simulink model "PV1"  (R2024b)
settings: Solver=ode4  StartTime=0.0  StopTime=100  FixedStep=0.00002  RelTol=1e-3
undefined symbols (not defined in the file): Ion, Lithium
libraries: spsSeriesRLCBranchLib x10, spsDiodeLib x3, spsMosfetLib x3, simulink x3, spsVoltageMeasurementLib x3, spsPVArrayLib x3, spsBatteryLib x1, spspowerguiLib x1
settings Model: Creator=Admin  LastModifiedBy=govin
settings RTWCC: GPUComputeCapability=3.5

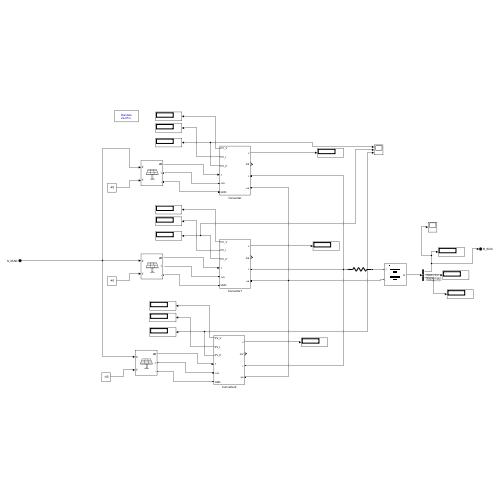
[thumbnail: Simulink's stored preview of the top-level diagram]
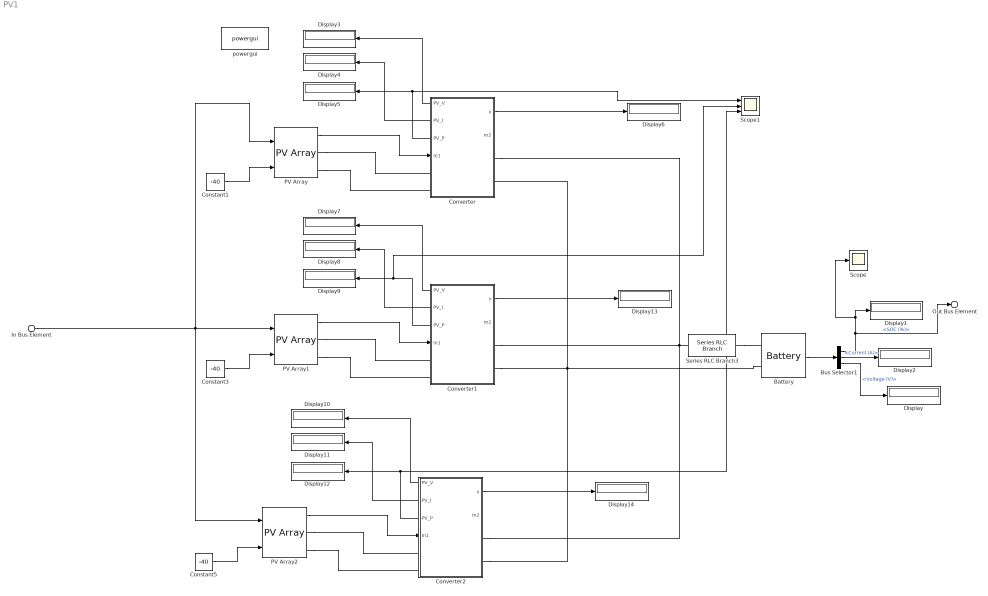
== system PV1 ==
  In Bus Element : Inport  PortName=S_IRAD
  Battery : spsBatteryLib/Battery  BatType=Lithium-Ion  NomV=8.4  NomQ=8  SOC=30  Batt_Tr=1  PresetModel=on  MaxQ=8  MinV=6.3  FullV=9.7775  Dis_rate=3.4783  R=0.0105  Normal_OP=7.2348  expZone="[9.0752     0.39304]"
  Bus Selector1 : BusSelector  OutputSignals=SOC (%),Current (A),Voltage (V)
  Constant1 : Constant  Value=-40
  Constant3 : Constant  Value=-40
  Constant5 : Constant  Value=-40
  Converter : Subsystem
      settings: PortSchema="{\"entries\":[{\"content\":{\"sides\":[{\"content\":{\"connectorIds\":[\"Out3\",\"Out4\",\"Out5\",\"In1\",\"LConn1\",\"LConn2\"]},\"type\":\"ConnectorPlacement.EquallySpacedRectSide\",\"uuid\":\"a132338a-6d9d-431e-bfe8-8757d124dffa\"},{\"content\":{\"connectorIds\":[\"Out1\",\"Out2\",\"RConn1\",\"RConn2\"],\"side\":\"RIGHT\"},\"type\":\"ConnectorPlacement.EquallySpacedRectSide\",\"uuid\":\"d50e3670-6251-4d2a-bf58-0033f338dba0\"},{\"content\":{\"side\":\"TOP\"},\"type\":\"ConnectorPlacement.EquallySpacedRectSide\",\"uuid\":\"35bc6587-48f1-421a-8d61-ff55cf247e3f\"}]},\"type\":\"ConnectorPlacement.EquallySpacedConnector\",\"uuid\":\"b4d66b82-5386-42ac-acc1-5dbc35c09c36\"}],\"packageUris\":[\"http://schema.mathworks.com/mf0/Connector/R2020b\"],\"version\":\"1.0\"}"
  Converter1 : Subsystem
      settings: PortSchema="{\"entries\":[{\"content\":{\"sides\":[{\"content\":{\"connectorIds\":[\"Out3\",\"Out4\",\"Out5\",\"In1\",\"LConn1\",\"LConn2\"]},\"type\":\"ConnectorPlacement.EquallySpacedRectSide\",\"uuid\":\"a132338a-6d9d-431e-bfe8-8757d124dffa\"},{\"content\":{\"connectorIds\":[\"Out1\",\"Out2\",\"RConn1\",\"RConn2\"],\"side\":\"RIGHT\"},\"type\":\"ConnectorPlacement.EquallySpacedRectSide\",\"uuid\":\"d50e3670-6251-4d2a-bf58-0033f338dba0\"},{\"content\":{\"side\":\"TOP\"},\"type\":\"ConnectorPlacement.EquallySpacedRectSide\",\"uuid\":\"35bc6587-48f1-421a-8d61-ff55cf247e3f\"}]},\"type\":\"ConnectorPlacement.EquallySpacedConnector\",\"uuid\":\"b4d66b82-5386-42ac-acc1-5dbc35c09c36\"}],\"packageUris\":[\"http://schema.mathworks.com/mf0/Connector/R2020b\"],\"version\":\"1.0\"}"
  Converter2 : Subsystem
      settings: PortSchema="{\"entries\":[{\"content\":{\"sides\":[{\"content\":{\"connectorIds\":[\"Out3\",\"Out4\",\"Out5\",\"In1\",\"LConn1\",\"LConn2\"]},\"type\":\"ConnectorPlacement.EquallySpacedRectSide\",\"uuid\":\"a132338a-6d9d-431e-bfe8-8757d124dffa\"},{\"content\":{\"connectorIds\":[\"Out1\",\"Out2\",\"RConn1\",\"RConn2\"],\"side\":\"RIGHT\"},\"type\":\"ConnectorPlacement.EquallySpacedRectSide\",\"uuid\":\"d50e3670-6251-4d2a-bf58-0033f338dba0\"},{\"content\":{\"side\":\"TOP\"},\"type\":\"ConnectorPlacement.EquallySpacedRectSide\",\"uuid\":\"35bc6587-48f1-421a-8d61-ff55cf247e3f\"}]},\"type\":\"ConnectorPlacement.EquallySpacedConnector\",\"uuid\":\"b4d66b82-5386-42ac-acc1-5dbc35c09c36\"}],\"packageUris\":[\"http://schema.mathworks.com/mf0/Connector/R2020b\"],\"version\":\"1.0\"}"
  Display{,1..14} (15 alike) : Display
  PV Array : spsPVArrayLib/PV Array  Npar=1  Nser=1  PlotType=array @ 25 deg.C & specified irradiances  S_vec="[ 1000  500  100 ]"  Temp_C_vec="[ 45 25  ]"  ModuleName=User-defined  PlotWhenSelected=off  Pm=8.6265  Ncell=7  Voc=19.25  Isc=0.521  Vm=17.15  Im=0.503  beta_Voc_pc=-0.59  alpha_Isc_pc=0.44  beta_Voc=-0.11357  alpha_Isc=0.0022924  IL=0.52617  I0=1.5749e-15  nI=3  Rsh=1905.5562  Rs=0.00066309  RobustModel=off  RobustCellTemperature=313.3991  BAL=on  Tc=1e-6  Tfilter=5e-5
  PV Array1 : spsPVArrayLib/PV Array  Npar=1  Nser=1  PlotType=array @ 25 deg.C & specified irradiances  S_vec="[ 1000  500  100 ]"  Temp_C_vec="[ 45 25  ]"  ModuleName=User-defined  PlotWhenSelected=off  Pm=7.3941  Ncell=7  Voc=16.5  Isc=0.521  Vm=14.7  Im=0.503  beta_Voc_pc=-0.59  alpha_Isc_pc=0.44  beta_Voc=-0.09735  alpha_Isc=0.0022924  IL=0.52104  I0=1.6325e-15  nI=2.8682  Rsh=1633.334  Rs=1.5927  RobustModel=off  RobustCellTemperature=313.3991  BAL=on  Tc=1e-6  Tfilter=5e-5
  PV Array2 : spsPVArrayLib/PV Array  Npar=1  Nser=1  PlotType=array @ 25 deg.C & specified irradiances  S_vec="[ 1000  500  100 ]"  Temp_C_vec="[ 45 25  ]"  ModuleName=User-defined  PlotWhenSelected=off  Pm=8.6265  Ncell=7  Voc=19.25  Isc=0.521  Vm=17.15  Im=0.503  beta_Voc_pc=-0.59  alpha_Isc_pc=0.44  beta_Voc=-0.11357  alpha_Isc=0.0022924  IL=0.52617  I0=1.5749e-15  nI=3  Rsh=1905.5562  Rs=0.00066309  RobustModel=off  RobustCellTemperature=313.3991  BAL=on  Tc=1e-6  Tfilter=5e-5
  Scope : Scope
  Scope1 : Scope  NumInputPorts=3
  Series RLC Branch3 : spsSeriesRLCBranchLib/Series RLC Branch  LConnTagsString=__new0  RConnTagsString=__new0  BranchType=R  Resistance=0.0001  Inductance=1e-3  SetiL0=off  InitialCurrent=0  Capacitance=0  Setx0=off  InitialVoltage=0  Measurements=None
  powergui : spspowerguiLib/powergui  Priority=1  SimulationMode=Discrete  SampleTime=0.00002  frequency=60  Iterations=50  frequencyindice=0  Pbase=100e6  ErrMax=1e-4  UnitsV=kV  UnitsW=MW  buscounter=0  FunctionMessages=off  echomessages=off  EnableUseOfTLC=off  CurrentSourceSwitches=off  DisableSnubberDevices=off  DisableRonSwitches=off  DisableVfSwitches=off  DisplayEquations=off  AutomaticDiscreteSolvers=off  SolverType=Tustin/Backward Euler (TBE)  Interpol=off  ExternalGateDelay=off  methode=off  Ts=100  x0status=blocks  SPID=on  SwTol=0  HookPort=off  NonlinearTolerance=1e-4  nMaxIteration=100  ContinueOnMaxIteration=off  RestoreLinks=warning  ResistiveCurrentMeasurement=off  Frange=[0:2:500]  Ylog=off  Xlog=on  ShowGrid=off  save=off  variable=ZData  structure=0  ZoomFFT=off  StartTime=0.0  cycles=1  DisplayStyle=1  fundamental=60  FreqAxis=off  MaxFrequency=1000  frequencyindicesteady=1  RmsSteady=1  display=off
  Out Bus Element : Outport  PortName=B_SOC
  wires:
  Constant1/1 -> PV Array/2
  Battery/1 -> Bus Selector1/1
  Bus Selector1/2 -> Display2/1  "<Current (A)>"
  Bus Selector1/1 -> Out Bus Element/1, Scope/1, Display1/1  "<SOC (%)>"
  Bus Selector1/3 -> Display/1  "<Voltage (V)>"
  Converter/1(v) -> Display6/1
  PV Array/1 -> Converter/1(In1)
  Converter/3(PV_V) -> Display3/1
  Converter/4(PV_I) -> Display4/1
  Converter/5(PV_P) -> Display5/1, Scope1/1
  Constant3/1 -> PV Array1/2
  Converter1/3(PV_V) -> Display7/1
  Converter1/1(v) -> Display13/1
  PV Array1/1 -> Converter1/1(In1)
  Converter1/4(PV_I) -> Display8/1
  Converter1/5(PV_P) -> Scope1/2, Display9/1
  Constant5/1 -> PV Array2/2
  Converter2/3(PV_V) -> Display10/1
  Converter2/1(v) -> Display14/1
  In Bus Element/1 -> PV Array/1, PV Array2/1, PV Array1/1
  PV Array2/1 -> Converter2/1(In1)
  Converter2/4(PV_I) -> Display11/1
  Converter2/5(PV_P) -> Scope1/3, Display12/1
  connections:
  Battery/LConn2 -- Converter/RConn2 -- Converter2/RConn2 -- Converter1/RConn2
  Converter/RConn1 -- Series RLC Branch3/LConn1 -- Converter2/RConn1 -- Converter1/RConn1
  PV Array/RConn1 -- Converter/LConn1
  PV Array/RConn2 -- Converter/LConn2
  PV Array1/RConn2 -- Converter1/LConn2
  PV Array1/RConn1 -- Converter1/LConn1
  PV Array2/RConn2 -- Converter2/LConn2
  PV Array2/RConn1 -- Converter2/LConn1
  Series RLC Branch3/RConn1 -- Battery/LConn1

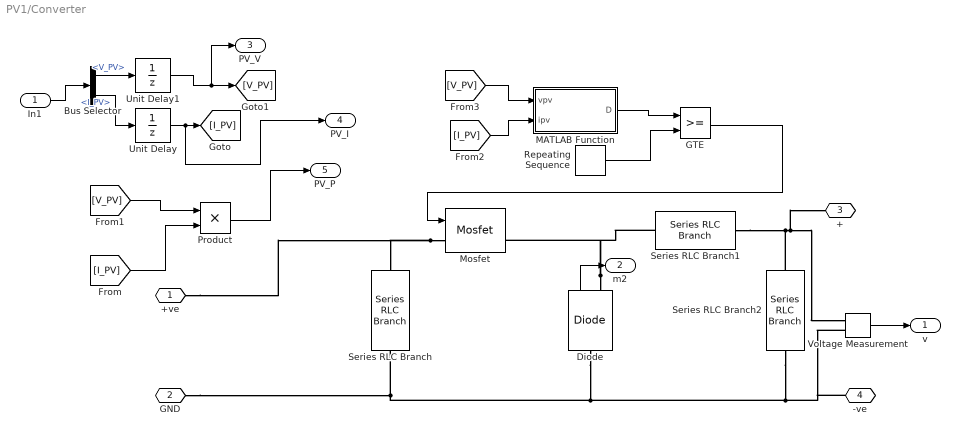
== system PV1/Converter ==
  In1 : Inport
  Bus Selector : BusSelector  OutputSignals=V_PV,I_PV
  Diode : spsDiodeLib/Diode  Ron=0.001  Lon=0  Vf=0.8  IC=0  UseSnubber=0  Rs=500  Cs=250e-9  Measurements=on
  GTE : RelationalOperator  OutDataTypeStr=boolean  RndMeth=Simplest  InputSameDT=off
  MATLAB Function : MATLAB Function  TreatAsAtomicUnit=on
  Mosfet : spsMosfetLib/Mosfet  Ron=0.1  Lon=0  Rd=0.01  Vfd=0  IC=0  Rs=1e5  Cs=inf  Measurements=on
  Product : Product
  Repeating Sequence : simulink/Sources/Repeating Sequence  rep_seq_t=[0 0.0002]  rep_seq_y=[0 1]
  Series RLC Branch : spsSeriesRLCBranchLib/Series RLC Branch  LConnTagsString=__new0  RConnTagsString=__new0  BranchType=RC  Resistance=0.0001  Inductance=1e-3  SetiL0=off  InitialCurrent=0  Capacitance=1000e-6  Setx0=off  InitialVoltage=0  Measurements=None
  Series RLC Branch1 : spsSeriesRLCBranchLib/Series RLC Branch  LConnTagsString=__new0  RConnTagsString=__new0  BranchType=L  Resistance=0.0001  Inductance=8.346e-3  SetiL0=off  InitialCurrent=0  Capacitance=1000e-6  Setx0=off  InitialVoltage=0  Measurements=None
  Series RLC Branch2 : spsSeriesRLCBranchLib/Series RLC Branch  LConnTagsString=__new0  RConnTagsString=__new0  BranchType=C  Resistance=0.0001  Inductance=0.865e-3  SetiL0=off  InitialCurrent=0  Capacitance=30.56e-6  Setx0=off  InitialVoltage=0  Measurements=None
  Unit Delay : UnitDelay  SampleTime=-1  HasFrameUpgradeWarning=on
  Unit Delay1 : UnitDelay  SampleTime=-1  HasFrameUpgradeWarning=on
  Voltage Measurement : spsVoltageMeasurementLib/Voltage Measurement  PhasorSimulation=off  OutputType=Complex  PSBequivalent=0
  +ve : PMIOPort  Side=Left
  GND : PMIOPort  Port=2  Side=Left
  + : PMIOPort  Port=3  Side=Right
  -ve : PMIOPort  Port=4  Side=Right
  v : Outport
  m2 : Outport  Port=2
  PV_V : Outport  Port=3
  PV_I : Outport  Port=4
  PV_P : Outport  Port=5
  wires:
  [V_PV] -> MATLAB Function/1(vpv)
  [I_PV] -> MATLAB Function/2(ipv)
  Repeating Sequence/1 -> GTE/2
  GTE/1 -> Mosfet/1
  MATLAB Function/1(D) -> GTE/1
  Diode/1 -> m2/1
  Voltage Measurement/1 -> v/1
  Bus Selector/2 -> Unit Delay/1  "<I_PV>"
  In1/1 -> Bus Selector/1
  Unit Delay/1 -> PV_I/1, [I_PV]
  Unit Delay1/1 -> PV_V/1, [V_PV]
  Bus Selector/1 -> Unit Delay1/1  "<V_PV>"
  [I_PV] -> Product/2
  [V_PV] -> Product/1
  Product/1 -> PV_P/1
  connections:
  Diode/LConn1 -- Voltage Measurement/LConn2 -- -ve/RConn1 -- Series RLC Branch2/RConn1 -- GND/RConn1 -- Series RLC Branch/RConn1
  Diode/RConn1 -- Series RLC Branch1/LConn1 -- Mosfet/RConn1
  Mosfet/LConn1 -- +ve/RConn1 -- Series RLC Branch/LConn1
  Series RLC Branch1/RConn1 -- Series RLC Branch2/LConn1 -- +/RConn1 -- Voltage Measurement/LConn1

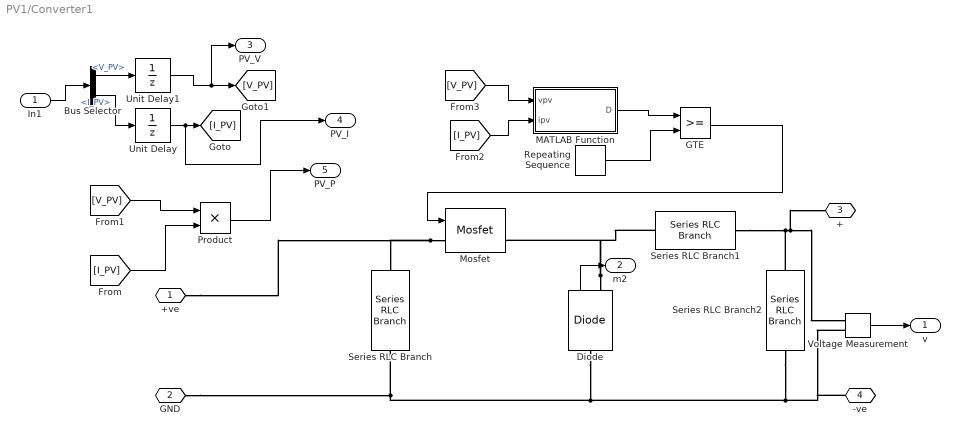
== system PV1/Converter1 ==
  In1 : Inport
  Bus Selector : BusSelector  OutputSignals=V_PV,I_PV
  Diode : spsDiodeLib/Diode  Ron=0.001  Lon=0  Vf=0.8  IC=0  UseSnubber=0  Rs=500  Cs=250e-9  Measurements=on
  GTE : RelationalOperator  OutDataTypeStr=boolean  RndMeth=Simplest  InputSameDT=off
  MATLAB Function : MATLAB Function  TreatAsAtomicUnit=on
  Mosfet : spsMosfetLib/Mosfet  Ron=0.1  Lon=0  Rd=0.01  Vfd=0  IC=0  Rs=1e5  Cs=inf  Measurements=on
  Product : Product
  Repeating Sequence : simulink/Sources/Repeating Sequence  rep_seq_t=[0 0.0002]  rep_seq_y=[0 1]
  Series RLC Branch : spsSeriesRLCBranchLib/Series RLC Branch  LConnTagsString=__new0  RConnTagsString=__new0  BranchType=RC  Resistance=0.0001  Inductance=1e-3  SetiL0=off  InitialCurrent=0  Capacitance=1000e-6  Setx0=off  InitialVoltage=0  Measurements=None
  Series RLC Branch1 : spsSeriesRLCBranchLib/Series RLC Branch  LConnTagsString=__new0  RConnTagsString=__new0  BranchType=L  Resistance=0.0001  Inductance=8.18e-3  SetiL0=off  InitialCurrent=0  Capacitance=1000e-6  Setx0=off  InitialVoltage=0  Measurements=None
  Series RLC Branch2 : spsSeriesRLCBranchLib/Series RLC Branch  LConnTagsString=__new0  RConnTagsString=__new0  BranchType=C  Resistance=0.0001  Inductance=0.865e-3  SetiL0=off  InitialCurrent=0  Capacitance=26.19e-6  Setx0=off  InitialVoltage=0  Measurements=None
  Unit Delay : UnitDelay  SampleTime=-1  HasFrameUpgradeWarning=on
  Unit Delay1 : UnitDelay  SampleTime=-1  HasFrameUpgradeWarning=on
  Voltage Measurement : spsVoltageMeasurementLib/Voltage Measurement  PhasorSimulation=off  OutputType=Complex  PSBequivalent=0
  +ve : PMIOPort  Side=Left
  GND : PMIOPort  Port=2  Side=Left
  + : PMIOPort  Port=3  Side=Right
  -ve : PMIOPort  Port=4  Side=Right
  v : Outport
  m2 : Outport  Port=2
  PV_V : Outport  Port=3
  PV_I : Outport  Port=4
  PV_P : Outport  Port=5
  wires:
  [V_PV] -> MATLAB Function/1(vpv)
  [I_PV] -> MATLAB Function/2(ipv)
  Repeating Sequence/1 -> GTE/2
  GTE/1 -> Mosfet/1
  MATLAB Function/1(D) -> GTE/1
  Diode/1 -> m2/1
  Voltage Measurement/1 -> v/1
  Bus Selector/2 -> Unit Delay/1  "<I_PV>"
  In1/1 -> Bus Selector/1
  Unit Delay/1 -> PV_I/1, [I_PV]
  Unit Delay1/1 -> PV_V/1, [V_PV]
  Bus Selector/1 -> Unit Delay1/1  "<V_PV>"
  [I_PV] -> Product/2
  [V_PV] -> Product/1
  Product/1 -> PV_P/1
  connections:
  Diode/LConn1 -- Voltage Measurement/LConn2 -- -ve/RConn1 -- Series RLC Branch2/RConn1 -- GND/RConn1 -- Series RLC Branch/RConn1
  Diode/RConn1 -- Series RLC Branch1/LConn1 -- Mosfet/RConn1
  Mosfet/LConn1 -- Series RLC Branch/LConn1 -- +ve/RConn1
  Series RLC Branch1/RConn1 -- Series RLC Branch2/LConn1 -- +/RConn1 -- Voltage Measurement/LConn1

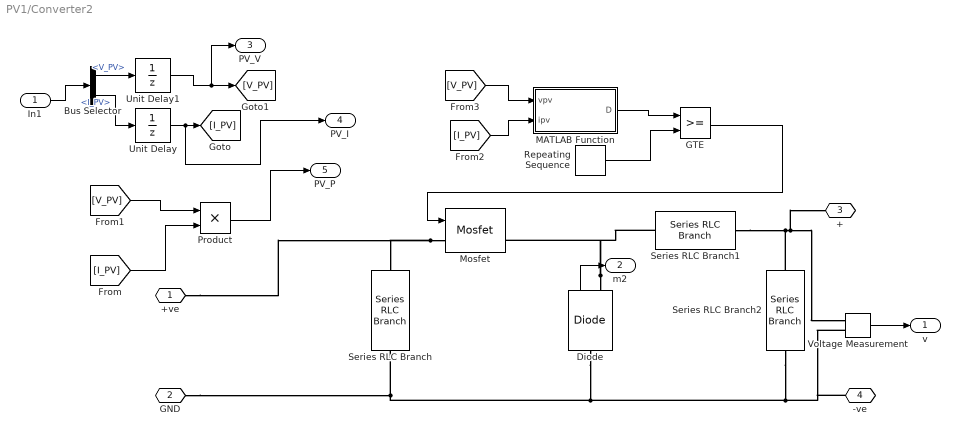
== system PV1/Converter2 ==
  In1 : Inport
  Bus Selector : BusSelector  OutputSignals=V_PV,I_PV
  Diode : spsDiodeLib/Diode  Ron=0.001  Lon=0  Vf=0.8  IC=0  UseSnubber=0  Rs=500  Cs=250e-9  Measurements=on
  GTE : RelationalOperator  OutDataTypeStr=boolean  RndMeth=Simplest  InputSameDT=off
  MATLAB Function : MATLAB Function  TreatAsAtomicUnit=on
  Mosfet : spsMosfetLib/Mosfet  Ron=0.1  Lon=0  Rd=0.01  Vfd=0  IC=0  Rs=1e5  Cs=inf  Measurements=on
  Product : Product
  Repeating Sequence : simulink/Sources/Repeating Sequence  rep_seq_t=[0 0.0002]  rep_seq_y=[0 1]
  Series RLC Branch : spsSeriesRLCBranchLib/Series RLC Branch  LConnTagsString=__new0  RConnTagsString=__new0  BranchType=RC  Resistance=0.0001  Inductance=1e-3  SetiL0=off  InitialCurrent=0  Capacitance=1000e-6  Setx0=off  InitialVoltage=0  Measurements=None
  Series RLC Branch1 : spsSeriesRLCBranchLib/Series RLC Branch  LConnTagsString=__new0  RConnTagsString=__new0  BranchType=L  Resistance=0.0001  Inductance=8.346e-3  SetiL0=off  InitialCurrent=0  Capacitance=1000e-6  Setx0=off  InitialVoltage=0  Measurements=None
  Series RLC Branch2 : spsSeriesRLCBranchLib/Series RLC Branch  LConnTagsString=__new0  RConnTagsString=__new0  BranchType=C  Resistance=0.0001  Inductance=0.865e-3  SetiL0=off  InitialCurrent=0  Capacitance=30.56e-6  Setx0=off  InitialVoltage=0  Measurements=None
  Unit Delay : UnitDelay  SampleTime=-1  HasFrameUpgradeWarning=on
  Unit Delay1 : UnitDelay  SampleTime=-1  HasFrameUpgradeWarning=on
  Voltage Measurement : spsVoltageMeasurementLib/Voltage Measurement  PhasorSimulation=off  OutputType=Complex  PSBequivalent=0
  +ve : PMIOPort  Side=Left
  GND : PMIOPort  Port=2  Side=Left
  + : PMIOPort  Port=3  Side=Right
  -ve : PMIOPort  Port=4  Side=Right
  v : Outport
  m2 : Outport  Port=2
  PV_V : Outport  Port=3
  PV_I : Outport  Port=4
  PV_P : Outport  Port=5
  wires:
  [V_PV] -> MATLAB Function/1(vpv)
  [I_PV] -> MATLAB Function/2(ipv)
  Repeating Sequence/1 -> GTE/2
  GTE/1 -> Mosfet/1
  MATLAB Function/1(D) -> GTE/1
  Diode/1 -> m2/1
  Voltage Measurement/1 -> v/1
  Bus Selector/2 -> Unit Delay/1  "<I_PV>"
  In1/1 -> Bus Selector/1
  Unit Delay/1 -> PV_I/1, [I_PV]
  Unit Delay1/1 -> PV_V/1, [V_PV]
  Bus Selector/1 -> Unit Delay1/1  "<V_PV>"
  [I_PV] -> Product/2
  [V_PV] -> Product/1
  Product/1 -> PV_P/1
  connections:
  Diode/LConn1 -- Voltage Measurement/LConn2 -- -ve/RConn1 -- Series RLC Branch2/RConn1 -- GND/RConn1 -- Series RLC Branch/RConn1
  Diode/RConn1 -- Series RLC Branch1/LConn1 -- Mosfet/RConn1
  Mosfet/LConn1 -- Series RLC Branch/LConn1 -- +ve/RConn1
  Series RLC Branch1/RConn1 -- Series RLC Branch2/LConn1 -- +/RConn1 -- Voltage Measurement/LConn1

== matlab function PV1/Converter/MATLAB Function ==
  data: vpv input; D output; ipv input
function D = MPPT_algorithm(vpv,ipv)
% Min and max value are used to limit duty between 0 and 1.06
Dmin=0;
Dmax=0.95;
Dinit=0.95;
DelD=0.0001;

persistent Vold Pold Dold;

datatype ='double';

if isempty(Vold)
    Vold=0;
    Pold=0;
    Dold=Dinit;
end

P= vpv*ipv; % power
dV= vpv - Vold; % difference between old and new voltage
dP= P - Pold;% difference between old and new power

% The algorithm in below search the dP/dV=0
% If the derivative equal to zero
% duty will not change if old and new power not equal &
% pv voltage bigger than 20V the algorithm will work
if dP ~= 0;
    if dP < 0;
        if dV < 0;
            D = Dold - DelD;
        else
            D = Dold + DelD;
        end
    else
        if dV < 0;
            D = Dold + DelD;
        else
            D = Dold - DelD;
        end
    end
else
    D=Dold;
end

%If limits the duty between min and max
if D >= Dmax || D <= Dmin;
    D=Dold;
end

Dold=D;
Vold=vpv;
Pold=P;

== matlab function PV1/Converter2/MATLAB Function ==
  data: vpv input; D output; ipv input
function D = MPPT_algorithm(vpv,ipv)
% Min and max value are used to limit duty between 0 and 1.06
Dmin=0;
Dmax=0.95;
Dinit=0.95;
DelD=0.0001;

persistent Vold Pold Dold;

datatype ='double';

if isempty(Vold)
    Vold=0;
    Pold=0;
    Dold=Dinit;
end

P= vpv*ipv; % power
dV= vpv - Vold; % difference between old and new voltage
dP= P - Pold;% difference between old and new power

% The algorithm in below search the dP/dV=0
% If the derivative equal to zero
% duty will not change if old and new power not equal &
% pv voltage bigger than 20V the algorithm will work
if dP ~= 0;
    if dP < 0;
        if dV < 0;
            D = Dold - DelD;
        else
            D = Dold + DelD;
        end
    else
        if dV < 0;
            D = Dold + DelD;
        else
            D = Dold - DelD;
        end
    end
else
    D=Dold;
end

%If limits the duty between min and max
if D >= Dmax || D <= Dmin;
    D=Dold;
end

Dold=D;
Vold=vpv;
Pold=P;

== matlab function PV1/Converter1/MATLAB Function ==
  data: vpv input; D output; ipv input
function D = MPPT_algorithm(vpv,ipv)
% Min and max value are used to limit duty between 0 and 1.06
Dmin=0;
Dmax=0.95;
Dinit=0.95;
DelD=0.0001;

persistent Vold Pold Dold;

datatype ='double';

if isempty(Vold)
    Vold=0;
    Pold=0;
    Dold=Dinit;
end

P= vpv*ipv; % power
dV= vpv - Vold; % difference between old and new voltage
dP= P - Pold;% difference between old and new power

% The algorithm in below search the dP/dV=0
% If the derivative equal to zero
% duty will not change if old and new power not equal &
% pv voltage bigger than 20V the algorithm will work
if dP ~= 0;
    if dP < 0;
        if dV < 0;
            D = Dold - DelD;
        else
            D = Dold + DelD;
        end
    else
        if dV < 0;
            D = Dold + DelD;
        else
            D = Dold - DelD;
        end
    end
else
    D=Dold;
end

%If limits the duty between min and max
if D >= Dmax || D <= Dmin;
    D=Dold;
end

Dold=D;
Vold=vpv;
Pold=P;
